simulink model "momentumBasedFlightSim"  (R2022a)
settings: Solver=FixedStepDiscrete  StartTime=0.0  StopTime=Config.simulationTime  FixedStep=Config.tStep  RelTol=1e-3
InitFcn:
  | cd(fileparts(which(bdroot)));
  | initMomentumBasedFlight;
StopFcn:
  | cd(fileparts(which(bdroot)));
  | stopMomentumBasedFlight;
undefined symbols (not defined in the file or in its folder): Config, DiscIntNeverNeededParam
libraries: WBToolboxLibrary x31, cstblocks x3, momentum_flight_control_sublib x2, thrust_estimation_sublib x1, jets_control x1
(part 1 of 2)
settings Model: NumberOfSteps=50  Creator=gnava  LastModifiedBy=gnava
settings SolverCC: AlgebraicLoopSolver=TrustRegion
settings DataIOCC: ReturnWorkspaceOutputs=off
settings OptimizationCC: BlockReduction=off  DefaultParameterBehavior=Inlined  BufferReuse=off
settings DebuggingCC: UnconnectedInputMsg=warning  UnconnectedOutputMsg=warning  UnconnectedLineMsg=warning  SFMachineParentedDataDiag=warning  ArithmeticOperatorsInVariantConditions=warning
settings SFSimCC: SimUseLocalCustomCode=off  CustomCodeUndefinedFunction=UseInterfaceOnly
settings RTWCC: RTWUseLocalCustomCode=off  DLArmComputeVersion=19.05

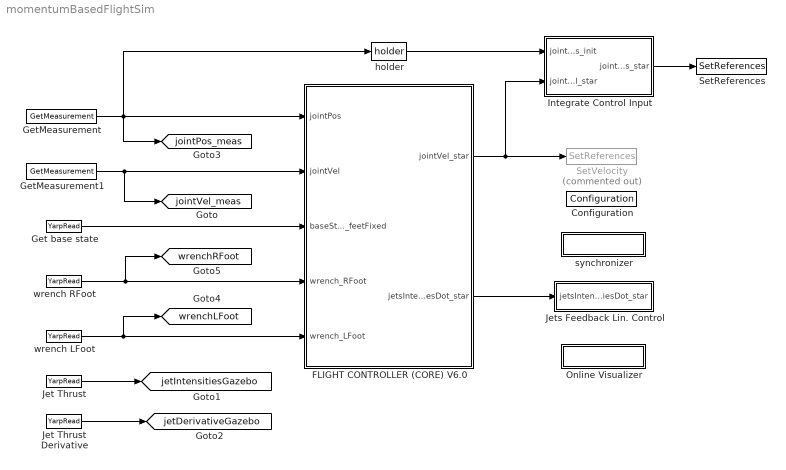
== system momentumBasedFlightSim ==
  Configuration : WBToolboxLibrary/Utilities/Configuration  ConfigSource=Workspace  ConfigObject='WBTConfigRobot'
      settings: SourceProductName=WholeBodyToolbox
  FLIGHT CONTROLLER (CORE) V6.0 : Subsystem
  Get base state : WBToolboxLibrary/Utilities/YarpRead  portName=Ports.BASE_STATE  signalSize=18  timeout=0.5  blocking=off  timestamp=off  autoconnect=on  errorOnConnection=on
      settings: SourceProductName=WholeBodyToolbox
  GetMeasurement : WBToolboxLibrary/States/GetMeasurement  measuredType=Joints Position
      settings: SourceProductName=WholeBodyToolbox
  GetMeasurement1 : WBToolboxLibrary/States/GetMeasurement  measuredType=Joints Velocity
      settings: SourceProductName=WholeBodyToolbox
  Integrate Control Input : Subsystem
  Jet Thrust : WBToolboxLibrary/Utilities/YarpRead  portName=Ports.THRUST  signalSize=4  timeout=0.5  blocking=off  timestamp=off  autoconnect=on  errorOnConnection=on
      settings: SourceProductName=WholeBodyToolbox
  Jet Thrust Derivative : WBToolboxLibrary/Utilities/YarpRead  portName=Ports.THRUST_DOT  signalSize=4  timeout=0.5  blocking=off  timestamp=off  autoconnect=on  errorOnConnection=off
      settings: SourceProductName=WholeBodyToolbox
  Jets Feedback Lin. Control : Subsystem
  Online Visualizer : Subsystem
      mask Display: disp("VISUALIZER")
  SetReferences : WBToolboxLibrary/Actuators/SetReferences  controlType=Position Direct  refSpeed=10*(pi/180)  refAcceleration=1000000*(pi/180)
      settings: SourceProductName=WholeBodyToolbox
  SetVelocity : WBToolboxLibrary/Actuators/SetReferences  Commented=on  controlType=Velocity  refSpeed=10*(pi/180)  refAcceleration=1000000*(pi/180)
      settings: SourceProductName=WholeBodyToolbox
  "holder " : WBToolboxLibrary/Utilities/holder 
      settings: SourceProductName=WholeBodyToolbox
  synchronizer : Subsystem
      mask Display: disp('SYNCHRONIZER')
  wrench LFoot : WBToolboxLibrary/Utilities/YarpRead  portName=Ports.WRENCH_LEFT_FOOT  signalSize=6  timeout=0.5  blocking=off  timestamp=off  autoconnect=on  errorOnConnection=on
      settings: SourceProductName=WholeBodyToolbox
  wrench RFoot : WBToolboxLibrary/Utilities/YarpRead  portName=Ports.WRENCH_RIGHT_FOOT  signalSize=6  timeout=0.5  blocking=off  timestamp=off  autoconnect=on  errorOnConnection=on
      settings: SourceProductName=WholeBodyToolbox
  tag scope: jetDerivativeGazebo=global, jetIntensitiesGazebo=global, jointPos_meas=global, jointVel_meas=global, wrenchLFoot=global, wrenchRFoot=global
  wires:
  GetMeasurement1/1 -> FLIGHT CONTROLLER (CORE) V6.0/2(jointVel), [jointVel_meas]
  wrench LFoot/1 -> FLIGHT CONTROLLER (CORE) V6.0/5(wrench_LFoot), [wrenchLFoot]
  wrench RFoot/1 -> FLIGHT CONTROLLER (CORE) V6.0/4(wrench_RFoot), [wrenchRFoot]
  "holder "/1 -> Integrate Control Input/1(jointPos_init)
  Integrate Control Input/1(jointPos_star) -> SetReferences/1
  Get base state/1 -> FLIGHT CONTROLLER (CORE) V6.0/3(baseState_feetFixed)
  GetMeasurement/1 -> FLIGHT CONTROLLER (CORE) V6.0/1(jointPos), [jointPos_meas], "holder "/1
  FLIGHT CONTROLLER (CORE) V6.0/2(jetsIntensitiesDot_star) -> Jets Feedback Lin. Control/1(jetsIntensitiesDot_star)
  Jet Thrust Derivative/1 -> [jetDerivativeGazebo]
  Jet Thrust/1 -> [jetIntensitiesGazebo]
  FLIGHT CONTROLLER (CORE) V6.0/1(jointVel_star) -> Integrate Control Input/2(jointVel_star), SetVelocity/1

== system momentumBasedFlightSim/FLIGHT CONTROLLER (CORE) V6.0 ==
  jointPos : Inport
  jointVel : Inport  Port=2
  baseState_feetFixed : Inport  Port=3
  wrench_RFoot : Inport  Port=4
  wrench_LFoot : Inport  Port=5
  Demux : Demux
  FLIGHT CONTROL : Subsystem
  Failure Detection : Subsystem
  STATE ESTIMATION : Subsystem
  Terminator : Terminator
  check failure detection : Scope  NumInputPorts=4
  jointVel_star : Outport  VectorParamsAs1DForOutWhenUnconnected=off
  jetsIntensitiesDot_star : Outport  Port=2  VectorParamsAs1DForOutWhenUnconnected=off
  wires:
  FLIGHT CONTROL/4(dynamics) -> STATE ESTIMATION/7(dynamics)
  jointPos/1 -> STATE ESTIMATION/1(jointPos)
  jointVel/1 -> STATE ESTIMATION/2(jointVel)
  baseState_feetFixed/1 -> STATE ESTIMATION/5(baseState_gazebo)
  STATE ESTIMATION/1(systemState) -> FLIGHT CONTROL/1(systemState), Failure Detection/1(systemState)
  wrench_RFoot/1 -> STATE ESTIMATION/3(wrench_RFoot)
  wrench_LFoot/1 -> STATE ESTIMATION/4(wrench_LFoot)
  [throttle] -> STATE ESTIMATION/6(Input throttle)
  FLIGHT CONTROL/1(jointVel_star) -> jointVel_star/1
  FLIGHT CONTROL/2(jetsIntensitiesDot_star) -> jetsIntensitiesDot_star/1, Failure Detection/2(jetsIntensitiesDot_star)
  FLIGHT CONTROL/3(jetsIntensities_des) -> Terminator/1
  Failure Detection/1(turbineStatus) -> Demux/1
  Demux/1 -> check failure detection/1  "lA"
  Demux/2 -> check failure detection/2  "rA"
  Demux/3 -> check failure detection/3  "lC"
  Demux/4 -> check failure detection/4  "rC"

== system momentumBasedFlightSim/Integrate Control Input ==
  jointPos_init : Inport
  jointVel_star : Inport  Port=2
  Discrete-Time Integrator : DiscreteIntegrator  InitialConditionSource=external  SampleTime=Config.tStep  ICPrevOutput=DiscIntNeverNeededParam  ICPrevScaledInput=DiscIntNeverNeededParam
  jointPos_star : Outport
  wires:
  Discrete-Time Integrator/1 -> jointPos_star/1
  jointVel_star/1 -> Discrete-Time Integrator/1
  jointPos_init/1 -> Discrete-Time Integrator/2

== system momentumBasedFlightSim/Jets Feedback Lin. Control ==
  jetsIntensitiesDot_star : Inport
  Bus Creator : BusCreator  Inputs=2
  Constant4 : Constant  Value=ones(4,1)*11
  Feedback Linearization Jets Control : jets_control/Feedback linearization 4-jets control  Conf=Config
      settings: SourceProductName=iRonCub Library
  Filter JetDerivative Desired : MATLAB Function  TreatAsAtomicUnit=on
  Logical Operator : Logic  Operator=NOT  AllPortsSameDT=off  OutDataTypeStr=boolean
  "ON_GAZEBO " : Constant  Value=Config.USE_JET_DYNAMICS
  SET THROTTLE : Subsystem
  SET_THRUST_DERIVATIVE : Subsystem
  tag scope: JetLog=global, throttle=global
  wires:
  Feedback Linearization Jets Control/1 -> [throttle], SET THROTTLE/1(throttle)
  Bus Creator/1 -> Feedback Linearization Jets Control/1
  [jetsIntensities] -> Filter JetDerivative Desired/1(jetIntensitiesEst), Bus Creator/1  "jetIntensitiesFiltered"
  [jetIntensitiesDot] -> Bus Creator/2  "jetDerivativesEst"
  "ON_GAZEBO "/1 -> SET THROTTLE/Enable, Logical Operator/1
  Logical Operator/1 -> SET_THRUST_DERIVATIVE/Enable
  Filter JetDerivative Desired/1(jetIntensitiesDerivativeDes) -> Feedback Linearization Jets Control/2
  jetsIntensitiesDot_star/1 -> SET_THRUST_DERIVATIVE/1(jetsIntensitiesDot_star), Filter JetDerivative Desired/2("jetIntensitiesDerivativeDes ")
  Constant4/1 -> [JetLog]

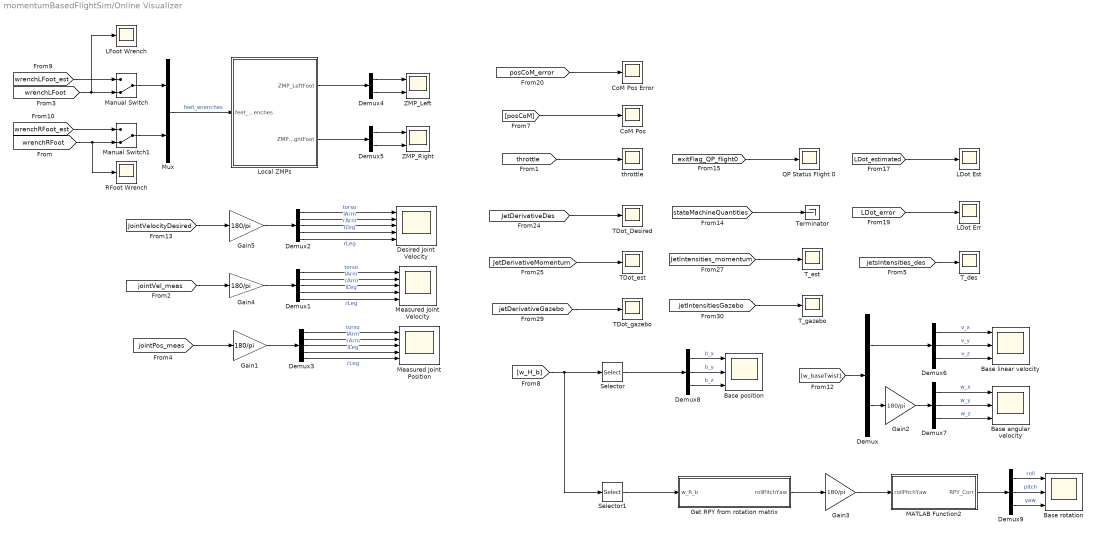
== system momentumBasedFlightSim/Online Visualizer ==
  Base angular velocity : Scope  NumInputPorts=3
  Base linear velocity : Scope  NumInputPorts=3
  Base position : Scope  NumInputPorts=3
  Base rotation : Scope  NumInputPorts=3
  CoM Pos : Scope
  CoM Pos Error : Scope
  Demux : Demux  Outputs=2
  Demux1 : Demux  Outputs=Config.numOfJointsForEachControlboard
  Demux2 : Demux  Outputs=Config.numOfJointsForEachControlboard
  Demux3 : Demux  Outputs=Config.numOfJointsForEachControlboard
  Demux4 : Demux  Outputs=2
  Demux5 : Demux  Outputs=2
  Demux{6..9} (4 alike) : Demux  Outputs=3
  Desired Joint Velocity : Scope  NumInputPorts=5
  Gain{1..5} (5 alike) : Gain  Gain=180/pi
  Get RPY from rotation matrix : MATLAB Function  TreatAsAtomicUnit=on
  LDot Err : Scope
  LDot Est : Scope
  LFoot Wrench : Scope
  Local ZMPs : Subsystem
  MATLAB Function2 : MATLAB Function  TreatAsAtomicUnit=on
  Manual Switch : ManualSwitch  CurrentSetting=0
  Manual Switch1 : ManualSwitch  CurrentSetting=0
  Measured Joint Position : Scope  NumInputPorts=5
  Measured Joint Velocity : Scope  NumInputPorts=5
  Mux : Mux  Inputs=2
  QP Status Flight 0 : Scope
  RFoot Wrench : Scope
  Selector : Selector  NumberOfDimensions=2  InputPortWidth=3  IndexOptions=Index vector (dialog),Index vector (dialog)  Indices=[1:3],4  OutputSizes=1,1
  Selector1 : Selector  NumberOfDimensions=2  InputPortWidth=3  IndexOptions=Index vector (dialog),Index vector (dialog)  Indices=[1:3],[1:3]  OutputSizes=1,1
  TDot_Desired : Scope
  TDot_est : Scope
  TDot_gazebo : Scope
  T_des : Scope
  T_est : Scope
  T_gazebo : Scope
  Terminator : Terminator
  ZMP_Left : Scope  NumInputPorts=2
  ZMP_Right : Scope  NumInputPorts=2
  throttle : Scope
  wires:
  Demux1/5 -> Measured Joint Velocity/5  "rLeg"
  Demux1/3 -> Measured Joint Velocity/3  "rArm"
  Demux1/1 -> Measured Joint Velocity/1  "torso"
  Demux1/4 -> Measured Joint Velocity/4  "lLeg"
  Gain4/1 -> Demux1/1
  [jointVel_meas] -> Gain4/1
  Demux1/2 -> Measured Joint Velocity/2  "lArm"
  Demux2/1 -> Desired Joint Velocity/1  "torso"
  Demux2/3 -> Desired Joint Velocity/3  "rArm"
  Demux2/4 -> Desired Joint Velocity/4  "lLeg"
  Demux2/5 -> Desired Joint Velocity/5  "rLeg"
  Demux2/2 -> Desired Joint Velocity/2  "lArm"
  Gain5/1 -> Demux2/1
  [throttle] -> throttle/1
  [JointVelocityDesired] -> Gain5/1
  [posCoM] -> CoM Pos/1
  Demux5/1 -> ZMP_Right/1
  Demux4/1 -> ZMP_Left/1
  Demux5/2 -> ZMP_Right/2
  Local ZMPs/2(ZMP_RightFoot) -> Demux5/1
  Demux4/2 -> ZMP_Left/2
  Local ZMPs/1(ZMP_LeftFoot) -> Demux4/1
  Mux/1 -> Local ZMPs/1(feet_wrenches)  "feet_wrenches"
  [wrenchLFoot_est] -> Manual Switch/1
  [wrenchLFoot] -> LFoot Wrench/1, Manual Switch/2
  [wrenchRFoot_est] -> Manual Switch1/1
  [wrenchRFoot] -> RFoot Wrench/1, Manual Switch1/2
  Manual Switch1/1 -> Mux/2
  Manual Switch/1 -> Mux/1
  [LDot_error] -> LDot Err/1
  [jetIntensitiesGazebo] -> T_gazebo/1
  [exitFlag_QP_flight0] -> QP Status Flight 0/1
  [stateMachineQuantities] -> Terminator/1
  [posCoM_error] -> CoM Pos Error/1
  [JetDerivativeMomentum] -> TDot_est/1
  [JetDerivativeDes] -> TDot_Desired/1
  [JetIntensities_momentum] -> T_est/1
  [jetDerivativeGazebo] -> TDot_gazebo/1
  [LDot_estimated] -> LDot Est/1
  Demux3/5 -> Measured Joint Position/5  "rLeg"
  Gain1/1 -> Demux3/1
  Demux3/4 -> Measured Joint Position/4  "lLeg"
  [jointPos_meas] -> Gain1/1
  Demux3/2 -> Measured Joint Position/2  "lArm"
  Demux3/3 -> Measured Joint Position/3  "rArm"
  Demux3/1 -> Measured Joint Position/1  "torso"
  [w_baseTwist] -> Demux/1
  Demux7/1 -> Base angular velocity/1  "w_x"
  Demux9/3 -> Base rotation/3  "yaw"
  Demux/2 -> Gain2/1
  Demux8/3 -> Base position/3  "b_z"
  Selector/1 -> Demux8/1
  Demux6/2 -> Base linear velocity/2  "v_y"
  Gain2/1 -> Demux7/1
  Demux8/1 -> Base position/1  "b_x"
  Demux9/1 -> Base rotation/1  "roll"
  Gain3/1 -> MATLAB Function2/1(rollPitchYaw)
  MATLAB Function2/1(RPY_Corr) -> Demux9/1
  Selector1/1 -> Get RPY from rotation matrix/1(w_R_b)
  Demux7/2 -> Base angular velocity/2  "w_y"
  Get RPY from rotation matrix/1(rollPitchYaw) -> Gain3/1
  Demux/1 -> Demux6/1
  Demux9/2 -> Base rotation/2  "pitch"
  Demux7/3 -> Base angular velocity/3  "w_z"
  Demux8/2 -> Base position/2  "b_y"
  Demux6/3 -> Base linear velocity/3  "v_z"
  [w_H_b] -> Selector1/1, Selector/1
  Demux6/1 -> Base linear velocity/1  "v_x"
  [jetsIntensities_des] -> T_des/1

== system momentumBasedFlightSim/synchronizer ==
  GAZEBO_SYNCHRONIZER : Subsystem
  Logical Operator : Logic  Operator=NOT  AllPortsSameDT=off  OutDataTypeStr=boolean
  "ON_GAZEBO " : Constant  Value=Config.ON_GAZEBO
  REAL_TIME_SYNCHRONIZER : Subsystem
  wires:
  Logical Operator/1 -> REAL_TIME_SYNCHRONIZER/Enable
  "ON_GAZEBO "/1 -> Logical Operator/1, GAZEBO_SYNCHRONIZER/Enable

== system momentumBasedFlightSim/FLIGHT CONTROLLER (CORE) V6.0/FLIGHT CONTROL ==
  systemState : Inport
  Bus Selector3 : BusSelector  OutputSignals=jetsIntensities_des
  Compute Global CoP : Subsystem
  Dynamics and Kinematics : momentum_flight_control_sublib/Dynamics and Kinematics  Parameter1=Config  Parameter2=Frames
      settings: SourceProductName=iRonCub Library
  Flight 0 Reference Generator : Subsystem
  Momentum-based Flight Control QP : Subsystem
  Terminator : Terminator
  Terminator1 : Terminator
  jointVel_star : Outport  VectorParamsAs1DForOutWhenUnconnected=off
  jetsIntensitiesDot_star : Outport  Port=2
  jetsIntensities_des : Outport  Port=3  VectorParamsAs1DForOutWhenUnconnected=off
  dynamics : Outport  Port=4
  wires:
  Compute Global CoP/2(global_cop_err_int) -> Terminator1/1
  Compute Global CoP/1(global_cop_err) -> Terminator/1
  Bus Selector3/1 -> jetsIntensities_des/1  "<jetsIntensities_des>"
  Dynamics and Kinematics/2 -> Flight 0 Reference Generator/2(dynamics), dynamics/1, Momentum-based Flight Control QP/5(dynamics)
  Momentum-based Flight Control QP/2(jetsIntensitiesDot_star) -> jetsIntensitiesDot_star/1
  Dynamics and Kinematics/1 -> Flight 0 Reference Generator/3(kinematics), Momentum-based Flight Control QP/4(kinematics)
  Flight 0 Reference Generator/2(feetContactIsActive) -> Momentum-based Flight Control QP/2(feetContactIsActive)
  systemState/1 -> Dynamics and Kinematics/1, Momentum-based Flight Control QP/3(systemState), Flight 0 Reference Generator/1(systemState), Compute Global CoP/1(systemState)
  Momentum-based Flight Control QP/1(jointVel_star) -> jointVel_star/1
  Flight 0 Reference Generator/1(gainsAndReferences) -> Momentum-based Flight Control QP/1(gainsAndReferences), Bus Selector3/1

== system momentumBasedFlightSim/FLIGHT CONTROLLER (CORE) V6.0/Failure Detection ==
  systemState : Inport
  jetsIntensitiesDot_star : Inport  Port=2
  Bus Selector3 : BusSelector  OutputSignals=jetsIntensities
  Clock : Clock
  Discrete-Time Integrator : DiscreteIntegrator  InitialConditionSource=external  SampleTime=Config.tStep  ICPrevOutput=DiscIntNeverNeededParam  ICPrevScaledInput=DiscIntNeverNeededParam
  Scope : Scope
  Scope1 : Scope
  Turbines Failure Detection : MATLAB Function  TreatAsAtomicUnit=on
  "holder " : WBToolboxLibrary/Utilities/holder 
      settings: SourceProductName=WholeBodyToolbox
  turbineStatus : Outport
  wires:
  Turbines Failure Detection/1(turbineStatus) -> turbineStatus/1
  systemState/1 -> Bus Selector3/1
  jetsIntensitiesDot_star/1 -> Discrete-Time Integrator/1
  Bus Selector3/1 -> Turbines Failure Detection/1(jetsIntensities), "holder "/1  "<jetsIntensities>"
  "holder "/1 -> Discrete-Time Integrator/2
  Clock/1 -> Turbines Failure Detection/3(t)
  Discrete-Time Integrator/1 -> Turbines Failure Detection/2(jetsIntensities_star)
  Turbines Failure Detection/2(T_err_avg) -> Scope/1
  Turbines Failure Detection/3(T_err) -> Scope1/1

== system momentumBasedFlightSim/FLIGHT CONTROLLER (CORE) V6.0/STATE ESTIMATION ==
  jointPos : Inport
  jointVel : Inport  Port=2
  wrench_RFoot : Inport  Port=3
  wrench_LFoot : Inport  Port=4
  baseState_gazebo : Inport  Port=5
  Input throttle : Inport  Port=6
  dynamics : Inport  Port=7
  CENTROIDAL MOMENTUM THRUST ESTIMATOR : Subsystem
  Get System State : momentum_flight_control_sublib/Get System State  Parameter1=Frames
      settings: SourceProductName=iRonCub Library
  Select Thrust Estimator : Subsystem
  systemState : Outport
  wires:
  Get System State/1 -> CENTROIDAL MOMENTUM THRUST ESTIMATOR/5(systemState), systemState/1
  jointPos/1 -> Get System State/1
  jointVel/1 -> Get System State/2
  wrench_LFoot/1 -> Get System State/5, CENTROIDAL MOMENTUM THRUST ESTIMATOR/4(wrench_LFoot)
  wrench_RFoot/1 -> Get System State/4, CENTROIDAL MOMENTUM THRUST ESTIMATOR/3(wrench_RFoot)
  Input throttle/1 -> CENTROIDAL MOMENTUM THRUST ESTIMATOR/2(Input throttle)
  dynamics/1 -> CENTROIDAL MOMENTUM THRUST ESTIMATOR/1(dynamics)
  Select Thrust Estimator/1(jetIntensities) -> Get System State/6
  Select Thrust Estimator/2(jetIntensitiesDot) -> Get System State/7
  baseState_gazebo/1 -> Get System State/3

== system momentumBasedFlightSim/Jets Feedback Lin. Control/SET THROTTLE ==
  throttle : Inport
  Enable : EnablePort
  Set Throttle : WBToolboxLibrary/Utilities/YarpWrite  portName=Ports.THROTTLE  autoconnect=on  errorOnConnection=on
      settings: SourceProductName=WholeBodyToolbox
  wires:
  throttle/1 -> Set Throttle/1

== system momentumBasedFlightSim/Jets Feedback Lin. Control/SET_THRUST_DERIVATIVE ==
  jetsIntensitiesDot_star : Inport
  Enable : EnablePort
  Constant : Constant  Value=-100
  Demux : Demux
  Manual Switch{,1..3} (4 alike) : ManualSwitch  CurrentSetting=0
  Mux : Mux
  Set Thrust Derivative : WBToolboxLibrary/Utilities/YarpWrite  portName=Ports.THRUST_RATIO  autoconnect=on  errorOnConnection=on
      settings: SourceProductName=WholeBodyToolbox
  wires:
  jetsIntensitiesDot_star/1 -> Demux/1
  Mux/1 -> Set Thrust Derivative/1
  Manual Switch3/1 -> Mux/4
  Manual Switch2/1 -> Mux/3
  Manual Switch1/1 -> Mux/2
  Manual Switch/1 -> Mux/1
  Demux/1 -> Manual Switch/2
  Demux/2 -> Manual Switch1/2
  Demux/3 -> Manual Switch2/2
  Demux/4 -> Manual Switch3/2
  Constant/1 -> Manual Switch3/1, Manual Switch2/1, Manual Switch1/1, Manual Switch/1

== system momentumBasedFlightSim/Online Visualizer/Local ZMPs ==
  feet_wrenches : Inport
  Demux1 : Demux  Outputs=3
  Demux2 : Demux  Outputs=3
  Divide{4..7} (4 alike) : Product  Inputs=*/
  Gain3 : Gain  Gain=-1
  Gain4 : Gain  Gain=-1
  Mux : Mux  Inputs=2
  Mux1 : Mux  Inputs=2
  fz taux tauy Left : Selector  InputPortWidth=12  IndexOptions=Index vector (dialog)  Indices=[3 4 5]  OutputSizes=1
  fz taux tauy Right : Selector  InputPortWidth=12  IndexOptions=Index vector (dialog)  Indices=[9 10 11]  OutputSizes=1
  ZMP_LeftFoot : Outport
  ZMP_RightFoot : Outport  Port=2
  wires:
  fz taux tauy Left/1 -> Demux1/1
  Demux1/1 -> Divide4/2, Divide5/2  "fzL"
  Divide7/1 -> Gain4/1
  Divide4/1 -> Mux/2
  Divide5/1 -> Gain3/1
  fz taux tauy Right/1 -> Demux2/1
  Demux2/1 -> Divide6/2, Divide7/2  "fzR"
  feet_wrenches/1 -> fz taux tauy Left/1, fz taux tauy Right/1
  Gain3/1 -> Mux/1
  Mux/1 -> ZMP_LeftFoot/1
  Divide6/1 -> Mux1/2
  Gain4/1 -> Mux1/1
  Mux1/1 -> ZMP_RightFoot/1
  Demux1/2 -> Divide4/1  "tauxL"
  Demux1/3 -> Divide5/1  "tauyL"
  Demux2/2 -> Divide6/1  "tauxR"
  Demux2/3 -> Divide7/1  "tauyR"

== system momentumBasedFlightSim/synchronizer/GAZEBO_SYNCHRONIZER ==
  Enable : EnablePort
  Simulator Synchronizer : WBToolboxLibrary/Utilities/Simulator Synchronizer  period=Config.tStep  serverPortName='/clock/rpc'  clientPortName='/WBT_synchronizer/rpc:o'
      settings: SourceProductName=WholeBodyToolbox

== system momentumBasedFlightSim/synchronizer/REAL_TIME_SYNCHRONIZER ==
  Enable : EnablePort
  Real Time Synchronizer : WBToolboxLibrary/Utilities/Real Time Synchronizer  period=Config.tStep
      settings: SourceProductName=WholeBodyToolbox

== system momentumBasedFlightSim/FLIGHT CONTROLLER (CORE) V6.0/FLIGHT CONTROL/Compute Global CoP ==
  systemState : Inport
  Add : Sum
  Bus Selector4 : BusSelector  OutputSignals=w_H_b,jointPos,contactForces
  CoP_err : Scope
  CoP_err_int : Scope
  Compute global CoP : MATLAB Function  TreatAsAtomicUnit=on
  Discrete-Time Integrator2 : DiscreteIntegrator  SampleTime=-1  ICPrevOutput=DiscIntNeverNeededParam  ICPrevScaledInput=DiscIntNeverNeededParam
  ForwardKinematics : WBToolboxLibrary/Model/Kinematics/ForwardKinematics  frameName=Frames.LFOOT_FRAME
      settings: SourceProductName=WholeBodyToolbox
  ForwardKinematics1 : WBToolboxLibrary/Model/Kinematics/ForwardKinematics  frameName=Frames.RFOOT_FRAME
      settings: SourceProductName=WholeBodyToolbox
  Gain : Gain  Gain=[0.5 0.5 0]'
  Matrix Multiply : Product
  Matrix Multiply1 : Product
  Scope : Scope  NumInputPorts=2
  Selector1 : Selector  NumberOfDimensions=2  InputPortWidth=3  IndexOptions=Index vector (dialog),Index vector (dialog)  Indices=[1:3],4  OutputSizes=1,1
  Selector2 : Selector  NumberOfDimensions=2  InputPortWidth=3  IndexOptions=Index vector (dialog),Index vector (dialog)  Indices=[1:3],4  OutputSizes=1,1
  Sum : Sum  Inputs=+-
  To Workspace2 : ToWorkspace  VariableName=wrench_left_right_transformed  SaveFormat=Structure With Time  SampleTime=-1
  global_cop_err : Outport
  global_cop_err_int : Outport  Port=2
  wires:
  Gain/1 -> Scope/1, Sum/1  "desired global cop"
  Add/1 -> Gain/1
  Selector1/1 -> Add/2
  Selector2/1 -> Add/1
  Matrix Multiply1/1 -> CoP_err_int/1, global_cop_err_int/1
  Matrix Multiply/1 -> CoP_err/1, global_cop_err/1
  Bus Selector4/3 -> To Workspace2/1  "<contactForces>"
  Discrete-Time Integrator2/1 -> Matrix Multiply1/2
  Compute global CoP/2(robotOnGround) -> Matrix Multiply1/1, Matrix Multiply/1
  Compute global CoP/1(global_cop) -> Scope/2, Sum/2  "global_cop"
  Bus Selector4/1 -> ForwardKinematics1/1, ForwardKinematics/1  "<w_H_b>"
  Sum/1 -> Discrete-Time Integrator2/1, Matrix Multiply/2
  ForwardKinematics/1 -> Selector2/1, Compute global CoP/3(H_left)
  ForwardKinematics1/1 -> Selector1/1, Compute global CoP/4(H_right)
  Bus Selector4/2 -> ForwardKinematics1/2, ForwardKinematics/2  "<jointPos>"
  [wrench_LFoot] -> Compute global CoP/1(wrench_left)
  systemState/1 -> Bus Selector4/1
  [wrench_RFoot] -> Compute global CoP/2(wrench_right)

== system momentumBasedFlightSim/FLIGHT CONTROLLER (CORE) V6.0/FLIGHT CONTROL/Flight 0 Reference Generator ==
  systemState : Inport
  dynamics : Inport  Port=2
  kinematics : Inport  Port=3
  Bus Selector : BusSelector  OutputSignals=jointPos,w_H_b
  Clock : Clock
  Compute Gains And References : Subsystem
  ForwardKinematics : WBToolboxLibrary/Model/Kinematics/ForwardKinematics  frameName=Frames.COM_FRAME
      settings: SourceProductName=WholeBodyToolbox
  Selector : Selector  NumberOfDimensions=2  InputPortWidth=3  IndexOptions=Index vector (dialog),Index vector (dialog)  Indices=[1 2 3],4  OutputSizes=1,1
  Selector1 : Selector  NumberOfDimensions=2  InputPortWidth=3  IndexOptions=Index vector (dialog),Index vector (dialog)  Indices=[1 2 3],[1 2 3]  OutputSizes=1,1
  Take Off/Landing State Detector : Subsystem
  gainsAndReferences : Outport
  feetContactIsActive : Outport  Port=2  VectorParamsAs1DForOutWhenUnconnected=off
  wires:
  kinematics/1 -> Compute Gains And References/6(kinematics)
  dynamics/1 -> Compute Gains And References/7(dynamics)
  Compute Gains And References/2(feetContactIsActive) -> feetContactIsActive/1
  Bus Selector/2 -> Selector1/1, ForwardKinematics/1  "<w_H_b>"
  Selector1/1 -> Compute Gains And References/2(w_R_b)
  Selector/1 -> Compute Gains And References/3(posCoM)
  Bus Selector/1 -> Compute Gains And References/1(jointPos), ForwardKinematics/2  "<jointPos>"
  ForwardKinematics/1 -> Selector/1
  Take Off/Landing State Detector/1(stateMachineQuantities) -> Compute Gains And References/4(stateMachineQuantities)
  Clock/1 -> Compute Gains And References/5(time)
  systemState/1 -> Take Off/Landing State Detector/1(systemState), Bus Selector/1
  Compute Gains And References/1(gainsAndReferences) -> gainsAndReferences/1

== system momentumBasedFlightSim/FLIGHT CONTROLLER (CORE) V6.0/FLIGHT CONTROL/Momentum-based Flight Control QP ==
  gainsAndReferences : Inport
  feetContactIsActive : Inport  Port=2
  systemState : Inport  Port=3
  kinematics : Inport  Port=4
  dynamics : Inport  Port=5
  Compute QP Quantities : Subsystem
  Filtering and Saturations : Subsystem
  QP Flight 0 : Subsystem
  jetsIntensitiesDot_postural : Scope
  jointVel_star : Outport  VectorParamsAs1DForOutWhenUnconnected=off
  jetsIntensitiesDot_star : Outport  Port=2  VectorParamsAs1DForOutWhenUnconnected=off
  wires:
  Filtering and Saturations/2(jointVel_star_filt) -> jointVel_star/1
  Filtering and Saturations/1(jetsIntensitiesDot_star_filt) -> jetsIntensitiesDot_star/1
  QP Flight 0/2(jointVel_star_QP) -> Filtering and Saturations/2(jointVel_star_QP), Compute QP Quantities/7(jointVel_star_QP)
  Compute QP Quantities/8(jetsIntensitiesDot_star_postural) -> jetsIntensitiesDot_postural/1
  Compute QP Quantities/7(ub_A) -> QP Flight 0/7(ub_A)
  Compute QP Quantities/6(lb_A) -> QP Flight 0/6(lb_A)
  Compute QP Quantities/5(A_matrix) -> QP Flight 0/5(A_matrix)
  Compute QP Quantities/4(upperBoundQP) -> QP Flight 0/4(upperBoundQP)
  Compute QP Quantities/3(lowerBoundQP) -> QP Flight 0/3(lowerBoundQP)
  Compute QP Quantities/2(gVectorQP) -> QP Flight 0/2(gVectorQP)
  Compute QP Quantities/1(HessianMatrixQP) -> QP Flight 0/1(HessianMatrixQP)
  feetContactIsActive/1 -> Compute QP Quantities/5(feetContactIsActive)
  gainsAndReferences/1 -> Compute QP Quantities/4(gainsAndReferences)
  dynamics/1 -> Compute QP Quantities/3(dynamics)
  kinematics/1 -> Compute QP Quantities/2(kinematics)
  systemState/1 -> Compute QP Quantities/1(systemState)
  QP Flight 0/1(jetIntensitiesDot_star_QP) -> Compute QP Quantities/6(jetsIntensitiesDot_star_QP), Filtering and Saturations/1(jetsIntensitiesDot_star_QP)

== system momentumBasedFlightSim/FLIGHT CONTROLLER (CORE) V6.0/STATE ESTIMATION/CENTROIDAL MOMENTUM THRUST ESTIMATOR ==
  dynamics : Inport
  Input throttle : Inport  Port=2
  wrench_RFoot : Inport  Port=3
  wrench_LFoot : Inport  Port=4
  systemState : Inport  Port=5
  Thrust Estimator (CORE) : Subsystem
  tag scope: JetDerivativeMomentum=global, JetIntensities_momentum=global, wrenchLFoot_est=global, wrenchRFoot_est=global
  wires:
  Thrust Estimator (CORE)/2(jetDerivativeEstimated) -> [JetDerivativeMomentum]
  systemState/1 -> Thrust Estimator (CORE)/1(systemState)
  Input throttle/1 -> Thrust Estimator (CORE)/5(Input throttle)
  Thrust Estimator (CORE)/1(jetIntensityFiltered) -> [JetIntensities_momentum]
  dynamics/1 -> Thrust Estimator (CORE)/2(dynamics)
  Thrust Estimator (CORE)/4(RFootWrenchEstimated) -> [wrenchRFoot_est]
  Thrust Estimator (CORE)/3(LFootWrenchEstimated) -> [wrenchLFoot_est]
  wrench_LFoot/1 -> Thrust Estimator (CORE)/4(wrench_LFoot)
  wrench_RFoot/1 -> Thrust Estimator (CORE)/3(wrench_RFoot)

== system momentumBasedFlightSim/FLIGHT CONTROLLER (CORE) V6.0/STATE ESTIMATION/Select Thrust Estimator ==
  Constant : Constant  Value=Config.USE_THRUST_ESTIMATOR
  Switch : Switch  Criteria=u2 > Threshold  SaturateOnIntegerOverflow=off  InputSameDT=off
  Switch1 : Switch  Criteria=u2 > Threshold  SaturateOnIntegerOverflow=off  InputSameDT=off
  jetIntensities : Outport
  jetIntensitiesDot : Outport  Port=2
  wires:
  [jetDerivativeGazebo] -> Switch1/3
  [JetDerivativeMomentum] -> Switch1/1
  [JetIntensities_momentum] -> Switch/1
  Switch/1 -> jetIntensities/1
  Switch1/1 -> jetIntensitiesDot/1
  [jetIntensitiesGazebo] -> Switch/3
  Constant/1 -> Switch1/2, Switch/2

== system momentumBasedFlightSim/FLIGHT CONTROLLER (CORE) V6.0/FLIGHT CONTROL/Flight 0 Reference Generator/Compute Gains And References ==
  jointPos : Inport
  w_R_b : Inport  Port=2
  posCoM : Inport  Port=3
  stateMachineQuantities : Inport  Port=4
  time : Inport  Port=5
  kinematics : Inport  Port=6
  dynamics : Inport  Port=7
  Bus Creator : BusCreator  Inputs=7
  Bus Selector1 : BusSelector  OutputSignals=feetContactIsActive
  "CoM6D -> CoMXYZ5" : Selector  NumberOfDimensions=2  InputPortWidth=7  IndexOptions=Index vector (dialog),Index vector (dialog)  Indices=[1 2 3],[1]  OutputSizes=1,1
  Compute Gains : Subsystem
  Online Planner : Subsystem
  "holder " : WBToolboxLibrary/Utilities/holder 
      settings: SourceProductName=WholeBodyToolbox
  holder 1 : WBToolboxLibrary/Utilities/holder 
      settings: SourceProductName=WholeBodyToolbox
  holder 2 : WBToolboxLibrary/Utilities/holder 
      settings: SourceProductName=WholeBodyToolbox
  gainsAndReferences : Outport  VectorParamsAs1DForOutWhenUnconnected=off
  feetContactIsActive : Outport  Port=2  VectorParamsAs1DForOutWhenUnconnected=off
  tag scope: jetsIntensities_des=global, jointPos_des=global, posCoM_des=global, rot_vel_acc_jerk_base_des=global
  wires:
  dynamics/1 -> Online Planner/7(dynamics)
  kinematics/1 -> Online Planner/6(kinematics)
  Online Planner/4(jetsIntensities_des) -> Bus Creator/4, [jetsIntensities_des]  "jetsIntensities_des"
  Online Planner/1(jointPos_des) -> [jointPos_des], Bus Creator/1  "jointPos_des"
  holder 2/1 -> Online Planner/2(jointPos_0)
  posCoM/1 -> "holder "/1
  w_R_b/1 -> holder 1/1
  "holder "/1 -> Online Planner/4(posCoM_0)
  holder 1/1 -> Online Planner/5(w_R_b_0)
  Bus Selector1/1 -> feetContactIsActive/1, Online Planner/1(feetContactIsActive)  "<feetContactIsActive>"
  time/1 -> Online Planner/3(time)
  stateMachineQuantities/1 -> Bus Selector1/1
  jointPos/1 -> holder 2/1
  "CoM6D -> CoMXYZ5"/1 -> [posCoM_des]
  Online Planner/3(pos_vel_acc_jerk_CoM_des) -> "CoM6D -> CoMXYZ5"/1, Bus Creator/3  "pos_vel_acc_jerk_CoM_des"
  Online Planner/2(rot_vel_acc_jerk_base_des) -> [rot_vel_acc_jerk_base_des], Bus Creator/2  "rot_vel_acc_jerk_base_des"
  Compute Gains/2(KD_momentum) -> Bus Creator/6  "KD_momentum"
  Compute Gains/1(KP_momentum) -> Bus Creator/5  "KP_momentum"
  Compute Gains/3(KP_postural) -> Bus Creator/7  "KP_postural"
  Bus Creator/1 -> gainsAndReferences/1

== system momentumBasedFlightSim/FLIGHT CONTROLLER (CORE) V6.0/FLIGHT CONTROL/Flight 0 Reference Generator/Take Off//Landing State Detector ==
  systemState : Inport
  Bus Creator : BusCreator  Inputs=3
  Bus Selector : BusSelector  OutputSignals=contactForces
  Demux : Demux  Outputs=[6;6]
  MATLAB Function : MATLAB Function  TreatAsAtomicUnit=on
  stateMachineQuantities : Outport  VectorParamsAs1DForOutWhenUnconnected=off
  tag scope: stateMachineQuantities=global
  wires:
  Bus Creator/1 -> [stateMachineQuantities], stateMachineQuantities/1
  systemState/1 -> Bus Selector/1
  Demux/2 -> MATLAB Function/2(wrench_r)
  Demux/1 -> MATLAB Function/1(wrench_l)
  Bus Selector/1 -> Demux/1  "<contactForces>"
  MATLAB Function/1(feetContactIsActive) -> Bus Creator/1  "feetContactIsActive"
  MATLAB Function/2(robotIsLanded) -> Bus Creator/2  "robotIsLanded"
  MATLAB Function/3(oneFootIsInContact) -> Bus Creator/3  "oneFootIsInContact"

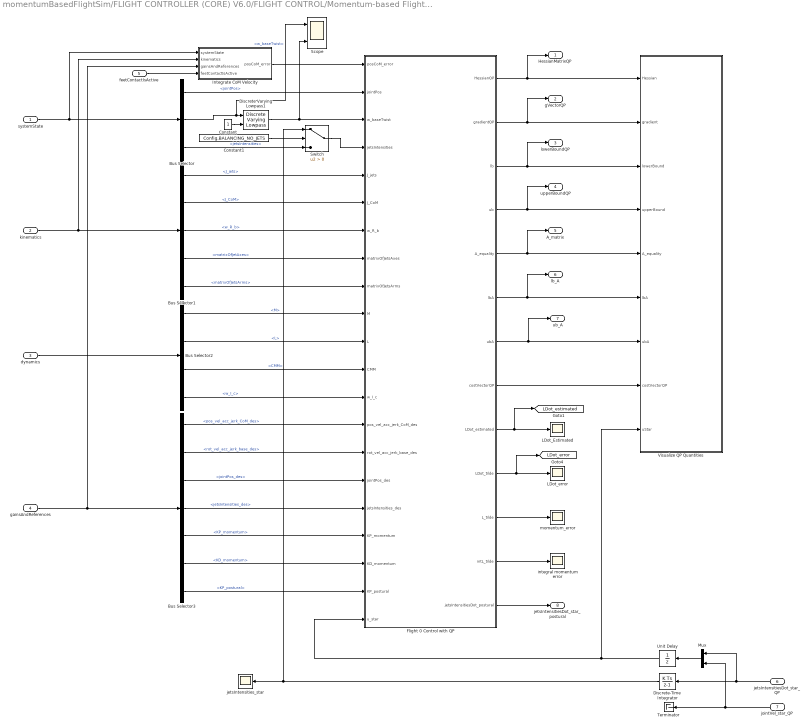
== system momentumBasedFlightSim/FLIGHT CONTROLLER (CORE) V6.0/FLIGHT CONTROL/Momentum-based Flight Control QP/Compute QP Quantities ==
  systemState : Inport
  kinematics : Inport  Port=2
  dynamics : Inport  Port=3
  gainsAndReferences : Inport  Port=4
  feetContactIsActive : Inport  Port=5
  jetsIntensitiesDot_star_QP : Inport  Port=6
  jointVel_star_QP : Inport  Port=7
  Bus Selector : BusSelector  OutputSignals=jointPos,w_baseTwist,jetsIntensities
  Bus Selector1 : BusSelector  OutputSignals=J_jets,J_CoM,w_R_b,matrixOfJetAxes,matrixOfJetsArms
  Bus Selector2 : BusSelector  OutputSignals=M,L,CMM,w_I_c
  Bus Selector3 : BusSelector  OutputSignals=pos_vel_acc_jerk_CoM_des,rot_vel_acc_jerk_base_des,jointPos_des,jetsIntensities_des,KP_momentum,KD_momentum,KP_postural
  Constant : Constant
  Constant1 : Constant  Value=Config.BALANCING_NO_JETS
  Discrete Varying Lowpass1 : cstblocks/Linear Parameter Varying/Discrete Varying Lowpass  N=2  w0=0  Ts=Config.tStep
      settings: SourceProductBaseCode=CT
  Discrete-Time Integrator : DiscreteIntegrator  InitialCondition=Config.inequalitiesQP.idleJetsInt  SampleTime=Config.tStep  ICPrevOutput=DiscIntNeverNeededParam  ICPrevScaledInput=DiscIntNeverNeededParam
  Flight 0 Control with QP : MATLAB Function  TreatAsAtomicUnit=on
  Integrate CoM Velocity : Subsystem
  LDot_Estimated : Scope
  LDot_error : Scope
  Mux : Mux  Inputs=2
  Scope : Scope  NumInputPorts=2
  Switch : Switch  Criteria=u2 > Threshold  SaturateOnIntegerOverflow=off  InputSameDT=off
  Terminator : Terminator
  Unit Delay : UnitDelay  SampleTime=-1  HasFrameUpgradeWarning=on
  Visualize QP Quantities : Subsystem
  integral momentum error : Scope
  jetsIntensities_star : Scope
  momentum_error : Scope
  HessianMatrixQP : Outport
  gVectorQP : Outport  Port=2
  lowerBoundQP : Outport  Port=3
  upperBoundQP : Outport  Port=4
  A_matrix : Outport  Port=5
  lb_A : Outport  Port=6
  ub_A : Outport  Port=7
  jetsIntensitiesDot_star_postural : Outport  Port=8  VectorParamsAs1DForOutWhenUnconnected=off
  tag scope: LDot_error=global, LDot_estimated=global
  wires:
  Flight 0 Control with QP/8(costVectorQP) -> Visualize QP Quantities/8(costVectorQP)
  Unit Delay/1 -> Visualize QP Quantities/9(uStar), Flight 0 Control with QP/21(u_star)
  jointVel_star_QP/1 -> Mux/2, Terminator/1
  Mux/1 -> Unit Delay/1
  Flight 0 Control with QP/13(jetsIntensitiesDot_postural) -> jetsIntensitiesDot_star_postural/1
  Flight 0 Control with QP/12(intL_tilde) -> integral momentum error/1
  Flight 0 Control with QP/11(L_tilde) -> momentum_error/1
  Flight 0 Control with QP/10(LDot_tilde) -> LDot_error/1, [LDot_error]
  Flight 0 Control with QP/9(LDot_estimated) -> [LDot_estimated], LDot_Estimated/1
  Flight 0 Control with QP/7(ubA) -> Visualize QP Quantities/7(ubA), ub_A/1
  Flight 0 Control with QP/6(lbA) -> lb_A/1, Visualize QP Quantities/6(lbA)
  Flight 0 Control with QP/5(A_equality) -> Visualize QP Quantities/5(A_equality), A_matrix/1
  Flight 0 Control with QP/4(ub) -> Visualize QP Quantities/4(upperBound), upperBoundQP/1
  Flight 0 Control with QP/3(lb) -> Visualize QP Quantities/3(lowerBound), lowerBoundQP/1
  Flight 0 Control with QP/2(gradientQP) -> Visualize QP Quantities/2(gradient), gVectorQP/1
  Flight 0 Control with QP/1(HessianQP) -> Visualize QP Quantities/1(Hessian), HessianMatrixQP/1
  Discrete-Time Integrator/1 -> Switch/1, jetsIntensities_star/1
  jetsIntensitiesDot_star_QP/1 -> Discrete-Time Integrator/1, Mux/1
  Bus Selector3/7 -> Flight 0 Control with QP/20(KP_postural)  "<KP_postural>"
  Bus Selector3/6 -> Flight 0 Control with QP/19(KD_momentum)  "<KD_momentum>"
  Bus Selector3/5 -> Flight 0 Control with QP/18(KP_momentum)  "<KP_momentum>"
  Bus Selector3/4 -> Flight 0 Control with QP/17(jetsIntensities_des)  "<jetsIntensities_des>"
  Bus Selector3/3 -> Flight 0 Control with QP/16(jointPos_des)  "<jointPos_des>"
  Bus Selector3/2 -> Flight 0 Control with QP/15(rot_vel_acc_jerk_base_des)  "<rot_vel_acc_jerk_base_des>"
  Bus Selector3/1 -> Flight 0 Control with QP/14(pos_vel_acc_jerk_CoM_des)  "<pos_vel_acc_jerk_CoM_des>"
  Bus Selector2/4 -> Flight 0 Control with QP/13(w_I_c)  "<w_I_c>"
  Bus Selector2/3 -> Flight 0 Control with QP/12(CMM)  "<CMM>"
  Bus Selector2/2 -> Flight 0 Control with QP/11(L)  "<L>"
  Bus Selector2/1 -> Flight 0 Control with QP/10(M)  "<M>"
  Bus Selector1/5 -> Flight 0 Control with QP/9(matrixOfJetsArms)  "<matrixOfJetsArms>"
  Bus Selector1/4 -> Flight 0 Control with QP/8(matrixOfJetsAxes)  "<matrixOfJetAxes>"
  Bus Selector1/3 -> Flight 0 Control with QP/7(w_R_b)  "<w_R_b>"
  Bus Selector1/2 -> Flight 0 Control with QP/6(J_CoM)  "<J_CoM>"
  Bus Selector1/1 -> Flight 0 Control with QP/5(J_jets)  "<J_jets>"
  Bus Selector/1 -> Flight 0 Control with QP/2(jointPos)  "<jointPos>"
  Bus Selector/2 -> Scope/1, Discrete Varying Lowpass1/1  "<w_baseTwist>"
  Switch/1 -> Flight 0 Control with QP/4(jetsIntensities)
  Integrate CoM Velocity/1(posCoM_error) -> Flight 0 Control with QP/1(posCoM_error)
  kinematics/1 -> Bus Selector1/1, Integrate CoM Velocity/2(kinematics)
  Bus Selector/3 -> Switch/3  "<jetsIntensities>"
  gainsAndReferences/1 -> Bus Selector3/1, Integrate CoM Velocity/3(gainsAndReferences)
  feetContactIsActive/1 -> Integrate CoM Velocity/4(feetContactIsActive)
  systemState/1 -> Bus Selector/1, Integrate CoM Velocity/1(systemState)
  dynamics/1 -> Bus Selector2/1
  Constant1/1 -> Switch/2
  Discrete Varying Lowpass1/1 -> Flight 0 Control with QP/3(w_baseTwist), Scope/2
  Constant/1 -> Discrete Varying Lowpass1/2

== system momentumBasedFlightSim/FLIGHT CONTROLLER (CORE) V6.0/FLIGHT CONTROL/Momentum-based Flight Control QP/Filtering and Saturations ==
  jetsIntensitiesDot_star_QP : Inport
  jointVel_star_QP : Inport  Port=2
  Filters on jetsIntensitiesDot : Subsystem
  Filters on jointVel : Subsystem
  jetsIntensitiesDot_star_filt : Outport
  jointVel_star_filt : Outport  Port=2  VectorParamsAs1DForOutWhenUnconnected=off
  tag scope: JetDerivativeDes=global, JointVelocityDesFlitered=global
  wires:
  Filters on jetsIntensitiesDot/1(jetsIntensitiesDot_star_filt) -> [JetDerivativeDes], jetsIntensitiesDot_star_filt/1
  Filters on jointVel/1(jointVel_star_filt) -> [JointVelocityDesFlitered], jointVel_star_filt/1
  jointVel_star_QP/1 -> Filters on jointVel/1(jointVel_star_QP)
  jetsIntensitiesDot_star_QP/1 -> Filters on jetsIntensitiesDot/1(jetsIntensitiesDot_star_QP)

== system momentumBasedFlightSim/FLIGHT CONTROLLER (CORE) V6.0/FLIGHT CONTROL/Momentum-based Flight Control QP/QP Flight 0 ==
  HessianMatrixQP : Inport
  gVectorQP : Inport  Port=2
  lowerBoundQP : Inport  Port=3
  upperBoundQP : Inport  Port=4
  A_matrix : Inport  Port=5
  lb_A : Inport  Port=6
  ub_A : Inport  Port=7
  Demux1 : Demux  Outputs=[4;Config.N_DOF]
  MatchSignalSizes : WBToolboxLibrary/Utilities/MatchSignalSizes
      settings: SourceProductName=WholeBodyToolbox
  OSQP : WBToolboxLibrary/Utilities/OSQP  lbA=on  ubA=on  lb=on  ub=on  computeObjVal=off  stopIfFails=on
      settings: SourceProductName=WholeBodyToolbox
  jetIntensitiesDot_star_QP : Outport
  jointVel_star_QP : Outport  Port=2
  tag scope: exitFlag_QP_flight0=global
  wires:
  MatchSignalSizes/1 -> Demux1/1
  A_matrix/1 -> OSQP/3
  lb_A/1 -> OSQP/4
  ub_A/1 -> OSQP/5
  upperBoundQP/1 -> OSQP/7
  lowerBoundQP/1 -> OSQP/6
  OSQP/2 -> [exitFlag_QP_flight0]
  gVectorQP/1 -> OSQP/2, MatchSignalSizes/1
  HessianMatrixQP/1 -> OSQP/1
  OSQP/1 -> MatchSignalSizes/2
  Demux1/1 -> jetIntensitiesDot_star_QP/1
  Demux1/2 -> jointVel_star_QP/1

== system momentumBasedFlightSim/FLIGHT CONTROLLER (CORE) V6.0/STATE ESTIMATION/CENTROIDAL MOMENTUM THRUST ESTIMATOR/Thrust Estimator (CORE) ==
  systemState : Inport
  dynamics : Inport  Port=2
  wrench_RFoot : Inport  Port=3
  wrench_LFoot : Inport  Port=4
  Input throttle : Inport  Port=5
  Bus Selector : BusSelector  OutputSignals=L
  Bus Selector1 : BusSelector  OutputSignals=jointPos,w_H_b
  Constant : Constant
  Constant1 : Constant  Value=0
  EKF-MOMENTUM_JET_FEET-CMM_FEET : thrust_estimation_sublib/For Simulation/EKF-MOMENTUM_JET_FEET-CMM_FEET  Ts=Config.tStep  Frames=Frames  T0=[0.0; 0.0; 0.0; 0.0]  dot_T0=[0.0; 0.0; 0.0; 0.0]  h0=[0.0; 0.0; 0.0; 0.0; 0.0; 0.0]  fLF0=[0.0; 0.0; 0.0; 0.0; 0.0; 0.0]  fRF0=[0.0; 0.0; 0.0; 0.0; 0.0; 0.0]  P0=blkdiag(eye(4)*1e1, eye(4)*1e1, eye(6)*1e1, eye(6)*1e1, eye(6)*1e1)  Q=blkdiag(eye(4)*1e1, eye(4)*1e1, eye(6)*1e1, eye(6)*1e1, eye(6)*1e1)  R=blkdiag(eye(6)*1e1, eye(6)*1e1, eye(6)*1e1)  jetC_P100=Config.jetC_P100  jetC_P220=Config.jetC_P220
      settings: SourceProductName=iRonCub Library
  Manual Switch : ManualSwitch
  Terminator : Terminator
  jetIntensityFiltered : Outport
  jetDerivativeEstimated : Outport  Port=2
  LFootWrenchEstimated : Outport  Port=3
  RFootWrenchEstimated : Outport  Port=4
  wires:
  EKF-MOMENTUM_JET_FEET-CMM_FEET/1 -> jetIntensityFiltered/1
  EKF-MOMENTUM_JET_FEET-CMM_FEET/2 -> jetDerivativeEstimated/1
  systemState/1 -> Bus Selector1/1
  dynamics/1 -> Bus Selector/1
  Input throttle/1 -> EKF-MOMENTUM_JET_FEET-CMM_FEET/1
  Bus Selector/1 -> EKF-MOMENTUM_JET_FEET-CMM_FEET/4  "<L>"
  Bus Selector1/2 -> EKF-MOMENTUM_JET_FEET-CMM_FEET/3  "<w_H_b>"
  wrench_RFoot/1 -> EKF-MOMENTUM_JET_FEET-CMM_FEET/6
  wrench_LFoot/1 -> EKF-MOMENTUM_JET_FEET-CMM_FEET/5
  Manual Switch/1 -> EKF-MOMENTUM_JET_FEET-CMM_FEET/7
  Constant1/1 -> Manual Switch/2
  Constant/1 -> Manual Switch/1
  EKF-MOMENTUM_JET_FEET-CMM_FEET/4 -> LFootWrenchEstimated/1
  EKF-MOMENTUM_JET_FEET-CMM_FEET/5 -> RFootWrenchEstimated/1
  EKF-MOMENTUM_JET_FEET-CMM_FEET/3 -> Terminator/1
  Bus Selector1/1 -> EKF-MOMENTUM_JET_FEET-CMM_FEET/2  "<jointPos>"

== system momentumBasedFlightSim/FLIGHT CONTROLLER (CORE) V6.0/FLIGHT CONTROL/Flight 0 Reference Generator/Compute Gains And References/Compute Gains ==
  Constant1 : Constant  Value=[Config.gains.momentum.KP_linear, Config.gains.momentum.KP_angular]
  Constant2 : Constant  Value=[Config.gains.momentum.KD_linear, Config.gains.momentum.KD_angular]
  Constant3 : Constant  Value=Config.gains.postural.KP
  Diagonalize : MATLAB Function  TreatAsAtomicUnit=on
  Diagonalize1 : MATLAB Function  TreatAsAtomicUnit=on
  Diagonalize2 : MATLAB Function  TreatAsAtomicUnit=on
  KP_momentum : Outport  VectorParamsAs1DForOutWhenUnconnected=off
  KD_momentum : Outport  Port=2  VectorParamsAs1DForOutWhenUnconnected=off
  KP_postural : Outport  Port=3  VectorParamsAs1DForOutWhenUnconnected=off
  tag scope: KD_momentum=global, KP_momentum=global, KP_postural=global
  wires:
  Diagonalize/1(K) -> KP_momentum/1
  Diagonalize1/1(K) -> KD_momentum/1
  Diagonalize2/1(K) -> KP_postural/1
  Constant1/1 -> [KP_momentum], Diagonalize/1(k)
  Constant2/1 -> [KD_momentum], Diagonalize1/1(k)
  Constant3/1 -> [KP_postural], Diagonalize2/1(k)

== system momentumBasedFlightSim/FLIGHT CONTROLLER (CORE) V6.0/FLIGHT CONTROL/Flight 0 Reference Generator/Compute Gains And References/Online Planner ==
  feetContactIsActive : Inport
  jointPos_0 : Inport  Port=2
  time : Inport  Port=3
  posCoM_0 : Inport  Port=4
  w_R_b_0 : Inport  Port=5
  kinematics : Inport  Port=6
  dynamics : Inport  Port=7
  Bus Selector1 : BusSelector  OutputSignals=matrixOfJetAxes,matrixOfJetsArms
  Bus Selector2 : BusSelector  OutputSignals=M
  Compute matrix Aj : MATLAB Function  TreatAsAtomicUnit=on
  Flight Planner - CoM and Base : MATLAB Function  TreatAsAtomicUnit=on
  Flight Planner - Joints and Thrusts : MATLAB Function  TreatAsAtomicUnit=on
  Selector : Selector  NumberOfDimensions=2  InputPortWidth=3  IndexOptions=Index vector (dialog),Index vector (dialog)  Indices=[1 2 3],3  OutputSizes=1,1
  Selector1 : Selector  NumberOfDimensions=2  InputPortWidth=3  IndexOptions=Index vector (dialog),Index vector (dialog)  Indices=1,1  OutputSizes=1,1
  Smooth CoM References : Subsystem
  Terminator : Terminator
  "holder " : WBToolboxLibrary/Utilities/holder 
      settings: SourceProductName=WholeBodyToolbox
  jointPos_des : Outport  VectorParamsAs1DForOutWhenUnconnected=off
  rot_vel_acc_jerk_base_des : Outport  Port=2  VectorParamsAs1DForOutWhenUnconnected=off
  pos_vel_acc_jerk_CoM_des : Outport  Port=3  VectorParamsAs1DForOutWhenUnconnected=off
  jetsIntensities_des : Outport  Port=4  VectorParamsAs1DForOutWhenUnconnected=off
  wires:
  Selector/1 -> Flight Planner - Joints and Thrusts/1(accCoM_des)
  Flight Planner - Joints and Thrusts/1(jetsIntensities_des) -> jetsIntensities_des/1
  Flight Planner - Joints and Thrusts/2(jointPos_des) -> jointPos_des/1
  Selector1/1 -> Flight Planner - Joints and Thrusts/2(m)
  Bus Selector2/1 -> Selector1/1  "<M>"
  "holder "/1 -> Flight Planner - Joints and Thrusts/4(Aj0)
  Compute matrix Aj/1(Aj) -> "holder "/1
  jointPos_0/1 -> Flight Planner - Joints and Thrusts/3(jointPos_0)
  Bus Selector1/2 -> Compute matrix Aj/2(matrixOfJetsArms)  "<matrixOfJetsArms>"
  Bus Selector1/1 -> Compute matrix Aj/1(matrixOfJetsAxes)  "<matrixOfJetAxes>"
  dynamics/1 -> Bus Selector2/1
  kinematics/1 -> Bus Selector1/1
  Flight Planner - CoM and Base/2(accCoM_gravity_ref) -> Smooth CoM References/2(accCoM_gravity_ref)
  Flight Planner - CoM and Base/1(posCoM_des) -> Smooth CoM References/1(posCoM_des)
  Smooth CoM References/1(pos_vel_acc_jerk_CoM_des) -> Selector/1, pos_vel_acc_jerk_CoM_des/1
  feetContactIsActive/1 -> Terminator/1
  posCoM_0/1 -> Flight Planner - CoM and Base/2(posCoM_0)
  Flight Planner - CoM and Base/3(rot_vel_acc_jerk_base_des) -> rot_vel_acc_jerk_base_des/1
  time/1 -> Flight Planner - CoM and Base/1(time)
  w_R_b_0/1 -> Flight Planner - CoM and Base/3(w_R_b_0)

== system momentumBasedFlightSim/FLIGHT CONTROLLER (CORE) V6.0/FLIGHT CONTROL/Momentum-based Flight Control QP/Compute QP Quantities/Integrate CoM Velocity ==
  systemState : Inport
  kinematics : Inport  Port=2
  gainsAndReferences : Inport  Port=3
  feetContactIsActive : Inport  Port=4
  Get CoM Position Error from Integral : Subsystem
  Get CoM Position Error from Integral but Only in Hovering : Subsystem
  Get CoM Position Error from Kinematics : Subsystem
  Select CoM Pos Error : Subsystem
  posCoM_error : Outport
  tag scope: posCoM_error=global
  wires:
  kinematics/1 -> Get CoM Position Error from Kinematics/1(kinematics), Get CoM Position Error from Integral but Only in Hovering/2(kinematics), Get CoM Position Error from Integral/1(kinematics)
  systemState/1 -> Get CoM Position Error from Integral but Only in Hovering/3(systemState), Get CoM Position Error from Integral/2(systemState)
  gainsAndReferences/1 -> Get CoM Position Error from Integral but Only in Hovering/4(gainsAndReferences), Get CoM Position Error from Kinematics/2(gainsAndReferences), Get CoM Position Error from Integral/3(gainsAndReferences)
  Select CoM Pos Error/1(posCoM_error) -> [posCoM_error], posCoM_error/1
  Get CoM Position Error from Integral but Only in Hovering/1(posCoM_error_fromInt_HoveringOnly) -> Select CoM Pos Error/2(posCoM_error_fromInt_HoveringOnly)
  Get CoM Position Error from Integral/1(posCoM_error_fromIntegral) -> Select CoM Pos Error/3(posCoM_error_fromIntegral)
  Get CoM Position Error from Kinematics/1(posCoM_error_fromKinematics) -> Select CoM Pos Error/4(posCoM_error_fromKinematics)
  feetContactIsActive/1 -> Select CoM Pos Error/1(feetContactIsActive), Get CoM Position Error from Integral but Only in Hovering/1(feetContactIsActive)

== system momentumBasedFlightSim/FLIGHT CONTROLLER (CORE) V6.0/FLIGHT CONTROL/Momentum-based Flight Control QP/Compute QP Quantities/Visualize QP Quantities ==
  Hessian : Inport
  gradient : Inport  Port=2
  lowerBound : Inport  Port=3
  upperBound : Inport  Port=4
  A_equality : Inport  Port=5
  lbA : Inport  Port=6
  ubA : Inport  Port=7
  costVectorQP : Inport  Port=8
  uStar : Inport  Port=9
  Cost Function : Subsystem
  Equality Constraints : Subsystem
  Input Boundaries : Subsystem
  Terminator : Terminator
  exitFlag_QP : Scope
  wires:
  [exitFlag_QP_flight0] -> exitFlag_QP/1
  upperBound/1 -> Input Boundaries/2(upperBound)
  lowerBound/1 -> Input Boundaries/1(lowerBound)
  costVectorQP/1 -> Cost Function/4(costVectorQP)
  gradient/1 -> Cost Function/3(gradient)
  Hessian/1 -> Cost Function/2(Hessian)
  ubA/1 -> Equality Constraints/1(upperBound_A)
  lbA/1 -> Terminator/1
  uStar/1 -> Cost Function/1(uStar), Equality Constraints/3(uStar), Input Boundaries/3(uStar)
  A_equality/1 -> Equality Constraints/2(A_equality)

== system momentumBasedFlightSim/FLIGHT CONTROLLER (CORE) V6.0/FLIGHT CONTROL/Momentum-based Flight Control QP/Filtering and Saturations/Filters on jetsIntensitiesDot ==
  jetsIntensitiesDot_star_QP : Inport
  Compare_filtered_jetIntensitiesDot : Scope  NumInputPorts=2
  Constant1 : Constant  Value=Config.FILTER_TDOT_AFTER_QP
  Constant2 : Constant  Value=Config.filter.cutOffFrequency
  Dead Zone : DeadZone  LowerValue=-Config.deadzone.jetsIntensitiesDot_deadzone  UpperValue=Config.deadzone.jetsIntensitiesDot_deadzone
  Discrete Varying Lowpass : cstblocks/Linear Parameter Varying/Discrete Varying Lowpass  N=2  w0=0  Ts=Config.tStep
      settings: SourceProductBaseCode=CT
  Saturation : Saturate  UpperLimit=Config.saturation.maxJetsIntVar  LowerLimit=-Config.saturation.maxJetsIntVar
  Switch : Switch  Criteria=u2 > Threshold  SaturateOnIntegerOverflow=off  InputSameDT=off
  jetsIntensitiesDot_star_filt : Outport
  wires:
  Constant1/1 -> Switch/2
  Constant2/1 -> Discrete Varying Lowpass/2
  Switch/1 -> jetsIntensitiesDot_star_filt/1
  Discrete Varying Lowpass/1 -> Dead Zone/1
  Saturation/1 -> Switch/1, Compare_filtered_jetIntensitiesDot/1
  Dead Zone/1 -> Saturation/1
  jetsIntensitiesDot_star_QP/1 -> Discrete Varying Lowpass/1, Switch/3, Compare_filtered_jetIntensitiesDot/2
